simulink model "trackVehicleNewVer6b_Encoders_DR_GNC2"  (R2018a)
settings: Solver=ode45  StartTime=0.0  StopTime=300  FixedStep=0.1  RelTol=1e-3  EnableMultiTasking=on
PreLoadFcn:
  | RTWConfigurationCB('preloadfcn', bdroot);
InitFcn:
  | parameterVehicle
  | parameterGNC
StartFcn:
  | start
StopFcn:
  | stop
  | myStopFcn2sim(xActEst,yActEst,X_array,Y_array,rp1,rp2)
values from neighbouring files (symbols this model uses):
  b = 0.32    [parameterVehicle.m]
  bDR = 1*b    [parameterGNC.m]
  dcArrayC = [-100  -60 0  60  100]    [parameterGNC.m]
  dcArrayL = [-100 ... (first row only)    [parameterVehicle.m]
  dcArrayR = [-100 ... (first row only)    [parameterVehicle.m]
  eTick = 4300    [parameterVehicle.m]
  eTickDR = eTick    [parameterGNC.m]
  KP2 = 2    [parameterGNC.m]
  rl = 0.87*rNominal    (= 0.05366131029)    [parameterVehicle.m]
  rNominal = 0.061679667    [parameterVehicle.m]
  rNominalDR = rNominal    [parameterGNC.m]
  rp1 = 0.5    [parameterGNC.m]
  rp2 = 0.3    [parameterGNC.m]
  rr = 1.00*rNominal    (= 0.061679667)    [parameterVehicle.m]
  Tau1 = 0.001    [parameterGNC.m]
  Tau2 = 0.01    [parameterGNC.m]
  TauEncoderDR = 0.001    [parameterGNC.m]
  thetaIC = 0*(pi/180)    (= 0)    [parameterVehicle.m]
  Tsample = 1/10    (= 0.1)    [parameterGNC.m]
  TsampleEncoder = 1/10    (= 0.1)    [parameterVehicle.m]
  TsampleEncoderDR = TsampleEncoder    [parameterGNC.m]
  Vcom = 3*VmaxDR/4    [parameterGNC.m]
  wArrayC = [-VmaxDR, -Vmin, 0,  Vmin, VmaxDR]./rNominalDR    [parameterGNC.m]
  wArrayL = [-1.622403101 ... (first row only)    [parameterVehicle.m]
  wArrayR = [-1.288449612 ... (first row only)    [parameterVehicle.m]
  X_array = [1 2]    [parameterGNC.m]
  xIC = 0    [parameterVehicle.m]
  Y_array = [0 0]    [parameterGNC.m]
  yIC = 0    [parameterVehicle.m]
undefined symbols (not defined in the file or in its folder): DiscIntNeverNeededParam
libraries: simulink x13, robotlib x8, aerolibanimutils x1
CloseFcn:
  | rtwprivate ssgencode ModelCloseRequest track_vehicle6_v2
settings Model: Creator=Dogan  LastModifiedBy=askar
settings DataIOCC: LimitDataPoints=on  SaveFormat=Array
settings OptimizationCC: ExpressionDepthLimit=2147483647  InitFltsAndDblsToZero=on  LifeSpan=inf
settings DebuggingCC: SaveWithParameterizedLinksMsg=none  UnderspecifiedInitializationDetection=Classic  MergeDetectMultiDrivingBlocksExec=none  SignalResolutionControl=TryResolveAllWithWarning  SolverPrmCheckMsg=warning  MultiTaskDSMMsg=warning  MultiTaskCondExecSysMsg=none  FcnCallInpInsideContextMsg=warning  StateNameClashWarn=warning  SFUnexpectedBacktrackingDiag=warning  SFNoUnconditionalDefaultTransitionDiag=warning  SFExecutionAtInitializationDiag=none
settings HardwareCC: ProdBitPerLong=64  ProdLargestAtomicFloat=None  ProdHWDeviceType=Intel->x86-64  TargetHWDeviceType=32-bit Generic
settings ModelReferenceCC: PropagateSignalLabelsOutOfModel=off
settings SFSimCC: SimParseCustomCode=off
settings RTWCC: Description=Generic Real-Time Target
settings CodeAppCC: GenerateComments=off  SimulinkBlockComments=off
settings GRTTargetCC: TargetLangStandard=C89/C90 (ANSI)  GeneratePreprocessorConditionals=Disable all
settings ConfigComp: CovMetricSettings=dw  CovHtmlReporting=on  CovSaveCumulativeToWorkspaceVar=on  CovSaveSingleToWorkspaceVar=on  CovExternalEMLEnable=off

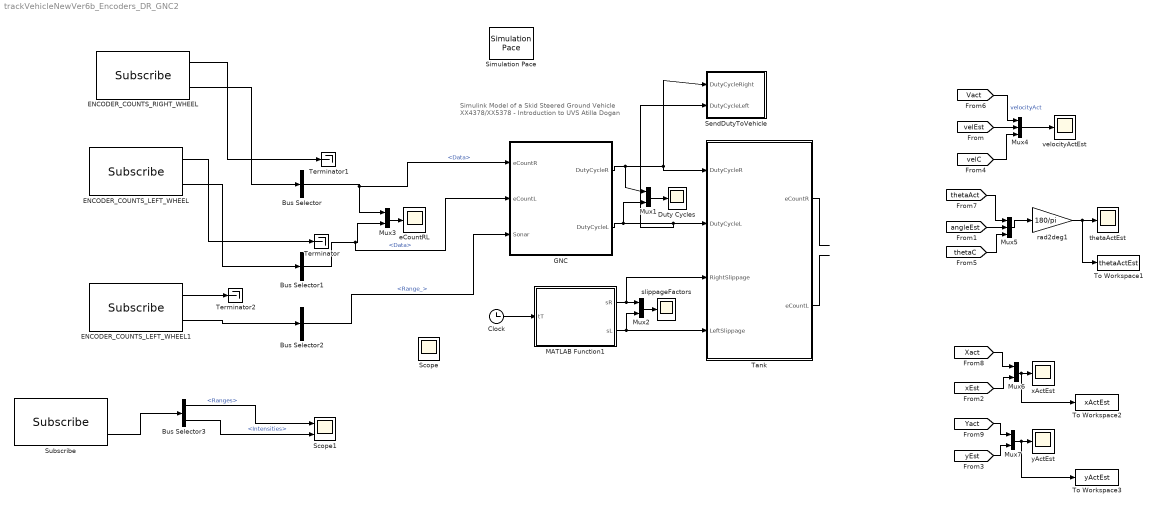
== system trackVehicleNewVer6b_Encoders_DR_GNC2 ==
  note: Simulink Model of a Skid Steered Ground Vehicle
      | XX4378/XX5378 - Introduction to UVS
      | Atilla Dogan
  Bus Selector : BusSelector  OutputSignals=Data
  Bus Selector1 : BusSelector  OutputSignals=Data
  Bus Selector2 : BusSelector  OutputSignals=Range_
  Bus Selector3 : BusSelector  OutputSignals=Ranges,Intensities
  Clock : Clock
  Duty Cycles : Scope
  ENCODER_COUNTS_LEFT_WHEEL : robotlib/Subscribe  SourceLibraryInfo=This block requires Robotics System Toolbox  topicSource=Select from ROS network  topic=/enco_L  messageType=std_msgs/Int16  sampleTime=-1  messageQueueLength=1
      settings: SourceProductBaseCode=RO
  ENCODER_COUNTS_LEFT_WHEEL1 : robotlib/Subscribe  SourceLibraryInfo=This block requires Robotics System Toolbox  topicSource=Select from ROS network  topic=/sonar  messageType=sensor_msgs/Range  sampleTime=-1  messageQueueLength=1
      settings: SourceProductBaseCode=RO
  ENCODER_COUNTS_RIGHT_WHEEL : robotlib/Subscribe  SourceLibraryInfo=This block requires Robotics System Toolbox  topicSource=Select from ROS network  topic=/enco_R  messageType=std_msgs/Int16  sampleTime=-1  messageQueueLength=1
      settings: SourceProductBaseCode=RO
  GNC : Subsystem
  MATLAB Function1 : MATLAB Function  TreatAsAtomicUnit=on
  Mux{1..3,6..7} (5 alike) : Mux  Inputs=2
  Mux4 : Mux  Inputs=3
  Mux5 : Mux  Inputs=3
  Scope : Scope
  Scope1 : Scope  NumInputPorts=2
  SendDutyToVehicle : Subsystem
  Simulation Pace : aerolibanimutils/Simulation Pace  SimulationPace=1  SleepMode=MATLAB Thread  OutputPaceError=off  SampleTime=1/30
  Subscribe : robotlib/Subscribe  SourceLibraryInfo=This block requires Robotics System Toolbox  topicSource=Select from ROS network  topic=/scan  messageType=sensor_msgs/LaserScan  sampleTime=-1  messageQueueLength=1
      settings: SourceProductBaseCode=RO
  Tank : Subsystem
  Terminator : Terminator
  Terminator1 : Terminator
  Terminator2 : Terminator
  To Workspace1 : ToWorkspace  VariableName=thetaActEst  SaveFormat=Structure With Time  SampleTime=-1
  To Workspace2 : ToWorkspace  VariableName=xActEst  SaveFormat=Structure With Time  SampleTime=-1
  To Workspace3 : ToWorkspace  VariableName=yActEst  SaveFormat=Structure With Time  SampleTime=-1
  eCountRL : Scope
  rad2deg1 : Gain  Gain=180/pi
  slippageFactors : Scope
  thetaActEst : Scope
  velocityActEst : Scope
  xActEst : Scope
  yActEst : Scope
  wires:
  MATLAB Function1/1(sR) -> Mux2/1, Tank/3(RightSlippage)
  MATLAB Function1/2(sL) -> Mux2/2, Tank/4(LeftSlippage)
  Clock/1 -> MATLAB Function1/1(tT)
  [Vact] -> Mux4/1  "velocityAct"
  GNC/1(DutyCycleR) -> Mux1/1, SendDutyToVehicle/1(DutyCycleRight), Tank/1(DutyCycleR)
  GNC/2(DutyCycleL) -> SendDutyToVehicle/2(DutyCycleLeft), Tank/2(DutyCycleL), Mux1/2
  Mux2/1 -> slippageFactors/1
  Mux1/1 -> Duty Cycles/1
  Tank/1(eCountR) -> ?
  Tank/2(eCountL) -> ?
  Mux4/1 -> velocityActEst/1
  [velEst] -> Mux4/2
  rad2deg1/1 -> To Workspace1/1, thetaActEst/1
  [thetaAct] -> Mux5/1
  Mux5/1 -> rad2deg1/1
  [angleEst] -> Mux5/2
  [Xact] -> Mux6/1
  [Yact] -> Mux7/1
  [xEst] -> Mux6/2
  Mux6/1 -> To Workspace2/1, xActEst/1
  Mux7/1 -> To Workspace3/1, yActEst/1
  [yEst] -> Mux7/2
  [velC] -> Mux4/3
  [thetaC] -> Mux5/3
  ENCODER_COUNTS_LEFT_WHEEL/1 -> Terminator/1
  ENCODER_COUNTS_RIGHT_WHEEL/2 -> Bus Selector/1
  ENCODER_COUNTS_RIGHT_WHEEL/1 -> Terminator1/1
  ENCODER_COUNTS_LEFT_WHEEL/2 -> Bus Selector1/1
  Bus Selector/1 -> GNC/1(eCountR), Mux3/1  "<Data>"
  Bus Selector1/1 -> GNC/2(eCountL), Mux3/2  "<Data>"
  Mux3/1 -> eCountRL/1
  ENCODER_COUNTS_LEFT_WHEEL1/2 -> Bus Selector2/1
  ENCODER_COUNTS_LEFT_WHEEL1/1 -> Terminator2/1
  Bus Selector2/1 -> GNC/3("Sonar ")  "<Range_>"
  Subscribe/2 -> Bus Selector3/1
  Bus Selector3/1 -> Scope1/1  "<Ranges>"
  Bus Selector3/2 -> Scope1/2  "<Intensities>"

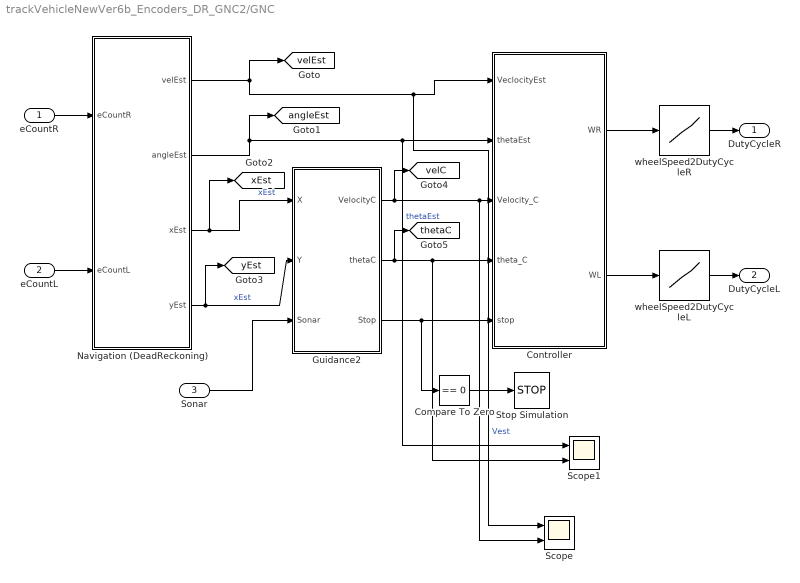
== system trackVehicleNewVer6b_Encoders_DR_GNC2/GNC ==
  eCountR : Inport
  eCountL : Inport  Port=2
  "Sonar " : Inport  Port=3
  Compare To Zero : simulink/Logic and Bit Operations/Compare To Zero  relop===  OutDataTypeStr=boolean
  Controller : Subsystem
  Guidance2 : Subsystem
  Navigation (DeadReckoning) : Subsystem
  Scope : Scope  NumInputPorts=2
  Scope1 : Scope  NumInputPorts=2
  Stop Simulation : Stop
  wheelSpeed2DutyCycleL : Lookup  InputValues=wArrayC  Table=dcArrayC  LookUpMeth=Interpolation-Use End Values
  wheelSpeed2DutyCycleR : Lookup  InputValues=wArrayC  Table=dcArrayC  LookUpMeth=Interpolation-Use End Values
  DutyCycleR : Outport
  DutyCycleL : Outport  Port=2
  tag scope: angleEst=global, thetaC=global, velC=global, velEst=global, xEst=global, yEst=global
  wires:
  Guidance2/3(Stop) -> Compare To Zero/1, Controller/5(stop)
  Controller/1(WR) -> wheelSpeed2DutyCycleR/1
  Navigation (DeadReckoning)/4(yEst) -> [yEst], Guidance2/2(Y)  "xEst"
  Navigation (DeadReckoning)/3(xEst) -> Guidance2/1(X), [xEst]  "xEst"
  Navigation (DeadReckoning)/2(angleEst) -> Scope1/1, Controller/2(thetaEst), [angleEst]  "thetaEst"
  Navigation (DeadReckoning)/1(velEst) -> Scope/1, Controller/1(VeclocityEst), [velEst]  "Vest"
  eCountL/1 -> Navigation (DeadReckoning)/2(eCountL)
  eCountR/1 -> Navigation (DeadReckoning)/1(eCountR)
  Guidance2/1(VelocityC) -> Scope/2, Controller/3(Velocity_C), [velC]
  Guidance2/2(thetaC) -> Scope1/2, Controller/4(theta_C), [thetaC]
  wheelSpeed2DutyCycleR/1 -> DutyCycleR/1
  Controller/2(WL) -> wheelSpeed2DutyCycleL/1
  wheelSpeed2DutyCycleL/1 -> DutyCycleL/1
  Compare To Zero/1 -> Stop Simulation/1
  "Sonar "/1 -> Guidance2/3("Sonar ")

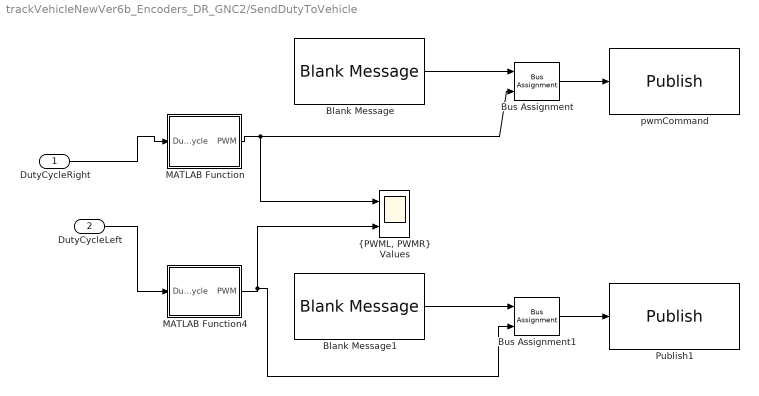
== system trackVehicleNewVer6b_Encoders_DR_GNC2/SendDutyToVehicle ==
  DutyCycleRight : Inport
  DutyCycleLeft : Inport  Port=2
  Blank Message : robotlib/Blank Message  SourceLibraryInfo=This block requires Robotics System Toolbox  messageType=std_msgs/Int16  SampleTime=inf
      settings: SourceProductBaseCode=RO
  Blank Message1 : robotlib/Blank Message  SourceLibraryInfo=This block requires Robotics System Toolbox  messageType=std_msgs/Int16  SampleTime=inf
      settings: SourceProductBaseCode=RO
  Bus Assignment : BusAssignment  AssignedSignals=Data
  Bus Assignment1 : BusAssignment  AssignedSignals=Data
  MATLAB Function : MATLAB Function  TreatAsAtomicUnit=on
  MATLAB Function4 : MATLAB Function  TreatAsAtomicUnit=on
  Publish1 : robotlib/Publish  SourceLibraryInfo=This block requires Robotics System Toolbox  topicSource=Select from ROS network  topic=/pwm_cmd_l  messageType=std_msgs/Int16  messageQueueLength=1
      settings: SourceProductBaseCode=RO
  pwmCommand : robotlib/Publish  SourceLibraryInfo=This block requires Robotics System Toolbox  topicSource=Select from ROS network  topic=/pwm_cmd_r  messageType=std_msgs/Int16  messageQueueLength=1
      settings: SourceProductBaseCode=RO
  "{PWML, PWMR} Values" : Scope  NumInputPorts=2
  wires:
  DutyCycleLeft/1 -> MATLAB Function4/1(DutyCycle)
  DutyCycleRight/1 -> MATLAB Function/1(DutyCycle)
  Blank Message/1 -> Bus Assignment/1
  MATLAB Function4/1(PWM) -> Bus Assignment1/2, "{PWML, PWMR} Values"/2
  MATLAB Function/1(PWM) -> Bus Assignment/2, "{PWML, PWMR} Values"/1
  Bus Assignment/1 -> pwmCommand/1
  Bus Assignment1/1 -> Publish1/1
  Blank Message1/1 -> Bus Assignment1/1

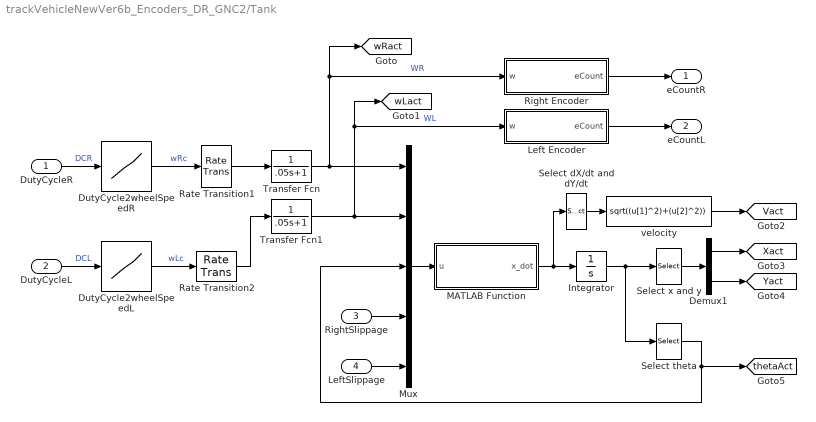
== system trackVehicleNewVer6b_Encoders_DR_GNC2/Tank ==
  DutyCycleR : Inport
  DutyCycleL : Inport  Port=2
  RightSlippage : Inport  Port=3
  LeftSlippage : Inport  Port=4
  Demux1 : Demux  Outputs=2
  DutyCycle2wheelSpeedL : Lookup  InputValues=dcArrayL  Table=wArrayL  LookUpMeth=Interpolation-Use End Values
  DutyCycle2wheelSpeedR : Lookup  InputValues=dcArrayR  Table=wArrayR  LookUpMeth=Interpolation-Use End Values
  Integrator : Integrator  InitialCondition=[xIC; yIC ; thetaIC]
  Left Encoder : Subsystem
  MATLAB Function : MATLAB Function  TreatAsAtomicUnit=on
  Mux : Mux  Inputs=5
  Rate Transition1 : RateTransition
  Rate Transition2 : RateTransition
  Right Encoder : Subsystem
  Select dX/dt and dY/dt : Selector  InputPortWidth=3  IndexOptions=Index vector (dialog)  Indices=[1 2]  OutputSizes=1
  Select theta : Selector  InputPortWidth=3  IndexOptions=Index vector (dialog)  Indices=3  OutputSizes=1
  Select x and y : Selector  InputPortWidth=3  IndexOptions=Index vector (dialog)  Indices=[1 2]  OutputSizes=1
  Transfer Fcn : TransferFcn  Denominator=[.05 1]
  Transfer Fcn1 : TransferFcn  Denominator=[.05 1]
  velocity : Fcn  Expr=sqrt((u[1]^2)+(u[2]^2))
  eCountR : Outport
  eCountL : Outport  Port=2
  tag scope: Vact=global, Xact=global, Yact=global, thetaAct=global, wLact=global, wRact=global
  wires:
  DutyCycleL/1 -> DutyCycle2wheelSpeedL/1  "DCL"
  DutyCycleR/1 -> DutyCycle2wheelSpeedR/1  "DCR"
  DutyCycle2wheelSpeedL/1 -> Rate Transition2/1  "wLc"
  DutyCycle2wheelSpeedR/1 -> Rate Transition1/1  "wRc"
  Rate Transition2/1 -> Transfer Fcn1/1
  Rate Transition1/1 -> Transfer Fcn/1
  Demux1/2 -> [Yact]
  Demux1/1 -> [Xact]
  Select x and y/1 -> Demux1/1
  velocity/1 -> [Vact]
  Select dX/dt and dY/dt/1 -> velocity/1
  MATLAB Function/1(x_dot) -> Integrator/1, Select dX/dt and dY/dt/1
  Select theta/1 -> [thetaAct], Mux/3
  Transfer Fcn/1 -> [wRact], Right Encoder/1(w), Mux/1  "WR"
  LeftSlippage/1 -> Mux/5
  RightSlippage/1 -> Mux/4
  Mux/1 -> MATLAB Function/1(u)
  Integrator/1 -> Select theta/1, Select x and y/1
  Transfer Fcn1/1 -> [wLact], Left Encoder/1(w), Mux/2  "WL"
  Left Encoder/1(eCount) -> eCountL/1
  Right Encoder/1(eCount) -> eCountR/1

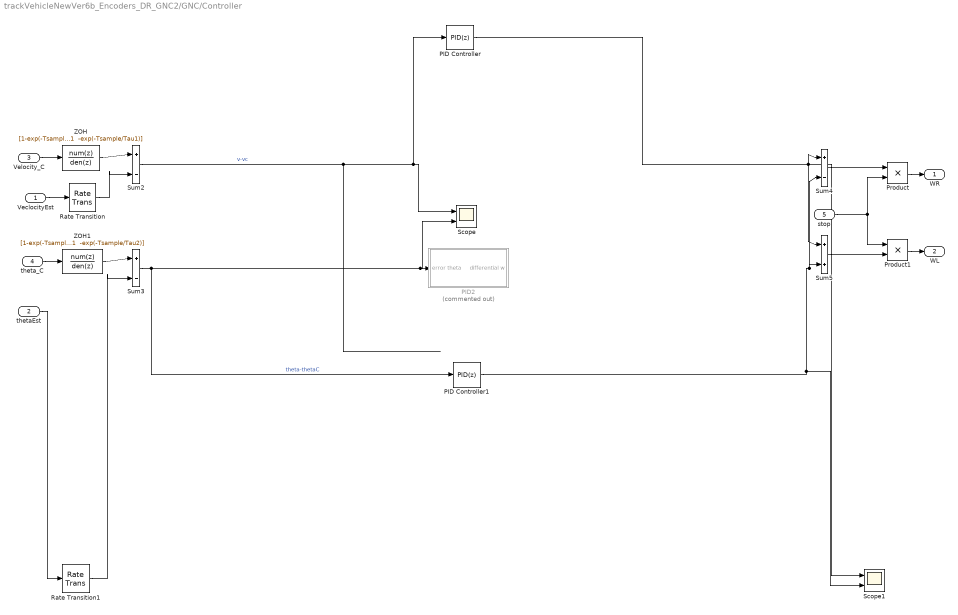
== system trackVehicleNewVer6b_Encoders_DR_GNC2/GNC/Controller ==
  VeclocityEst : Inport
  thetaEst : Inport  Port=2
  Velocity_C : Inport  Port=3
  theta_C : Inport  Port=4
  stop : Inport  Port=5
  PID Controller : simulink/Continuous/PID Controller  Controller=PID  TimeDomain=Discrete-time  SampleTime=-1  IntegratorMethod=Forward Euler  FilterMethod=Forward Euler  Form=Parallel  UseFilter=off  ControllerParametersSource=internal  P=2  I=7.0932  D=0.01  N=100  InitialConditionSource=internal  InitialConditionForIntegrator=0  InitialConditionForFilter=0  ExternalReset=none  LimitOutput=off  UpperSaturationLimit=inf  LowerSaturationLimit=-inf  LinearizeAsGain=on  AntiWindupMode=none  Kb=1  TrackingMode=off  Kt=1  PParamMin=[]  PParamMax=[]  IParamMin=[]  IParamMax=[]  DParamMin=[]  DParamMax=[]  NParamMin=[]  NParamMax=[]  KbParamMin=[]  KbParamMax=[]  KtParamMin=[]  KtParamMax=[]  POutMin=[]  POutMax=[]  IOutMin=[]  IOutMax=[]  DOutMin=[]  DOutMax=[]  NOutMin=[]  NOutMax=[]  KbOutMin=[]  KbOutMax=[]  KtOutMin=[]  KtOutMax=[]  IntegratorOutMin=[]  IntegratorOutMax=[]  FilterOutMin=[]  FilterOutMax=[]  SumOutMin=[]  SumOutMax=[]  SumI1OutMin=[]  SumI1OutMax=[]  SumI2OutMin=[]  SumI2OutMax=[]  SumI3OutMin=[]  SumI3OutMax=[]  SumDOutMin=[]  SumDOutMax=[]  SaturationOutMin=[]  SaturationOutMax=[]  IntegratorContinuousStateAttributes=''  IntegratorStateMustResolveToSignalObject=off  IntegratorRTWStateStorageClass=Auto  FilterContinuousStateAttributes=''  FilterStateMustResolveToSignalObject=off  FilterRTWStateStorageClass=Auto  DifferentiatorICPrevScaledInput=0  DifferentiatorOutMin=[]  DifferentiatorOutMax=[]  FilterDiffOutCoefMin=[]  FilterDiffOutCoefMax=[]  SumDenOutMin=[]  SumDenOutMax=[]  SumNumOutMin=[]  SumNumOutMax=[]  ReciprocalOutMin=[]  ReciprocalOutMax=[]  DivideOutMin=[]  DivideOutMax=[]  TunerSelectOption=Frequency Response Based
  PID Controller1 : simulink/Continuous/PID Controller  Controller=PID  TimeDomain=Discrete-time  SampleTime=-1  IntegratorMethod=Forward Euler  FilterMethod=Forward Euler  Form=Parallel  UseFilter=off  ControllerParametersSource=internal  P=6.4  I=1.2  D=1.8  N=100  InitialConditionSource=internal  InitialConditionForIntegrator=0  InitialConditionForFilter=0  ExternalReset=none  LimitOutput=off  UpperSaturationLimit=inf  LowerSaturationLimit=-inf  LinearizeAsGain=on  AntiWindupMode=none  Kb=1  TrackingMode=off  Kt=1  PParamMin=[]  PParamMax=[]  IParamMin=[]  IParamMax=[]  DParamMin=[]  DParamMax=[]  NParamMin=[]  NParamMax=[]  KbParamMin=[]  KbParamMax=[]  KtParamMin=[]  KtParamMax=[]  POutMin=[]  POutMax=[]  IOutMin=[]  IOutMax=[]  DOutMin=[]  DOutMax=[]  NOutMin=[]  NOutMax=[]  KbOutMin=[]  KbOutMax=[]  KtOutMin=[]  KtOutMax=[]  IntegratorOutMin=[]  IntegratorOutMax=[]  FilterOutMin=[]  FilterOutMax=[]  SumOutMin=[]  SumOutMax=[]  SumI1OutMin=[]  SumI1OutMax=[]  SumI2OutMin=[]  SumI2OutMax=[]  SumI3OutMin=[]  SumI3OutMax=[]  SumDOutMin=[]  SumDOutMax=[]  SaturationOutMin=[]  SaturationOutMax=[]  IntegratorContinuousStateAttributes=''  IntegratorStateMustResolveToSignalObject=off  IntegratorRTWStateStorageClass=Auto  FilterContinuousStateAttributes=''  FilterStateMustResolveToSignalObject=off  FilterRTWStateStorageClass=Auto  DifferentiatorICPrevScaledInput=0  DifferentiatorOutMin=[]  DifferentiatorOutMax=[]  FilterDiffOutCoefMin=[]  FilterDiffOutCoefMax=[]  SumDenOutMin=[]  SumDenOutMax=[]  SumNumOutMin=[]  SumNumOutMax=[]  ReciprocalOutMin=[]  ReciprocalOutMax=[]  DivideOutMin=[]  DivideOutMax=[]  TunerSelectOption=Frequency Response Based
  PID2 : Subsystem  Commented=on
  Product : Product  RndMeth=Zero
  Product1 : Product  RndMeth=Zero
  Rate Transition : RateTransition  Deterministic=off
  Rate Transition1 : RateTransition  Deterministic=off
  Scope : Scope  NumInputPorts=2
  Scope1 : Scope  NumInputPorts=2
  Sum2 : Sum  Inputs=|+|-|  SampleTime=Tsample
  Sum3 : Sum  Inputs=|+|-|  SampleTime=Tsample
  Sum4 : Sum  Inputs=+|-
  Sum5 : Sum  Inputs=+|+
  ZOH : DiscreteTransferFcn  Numerator=[1-exp(-Tsample/Tau1)]  Denominator="[1  -exp(-Tsample/Tau1)]"  SampleTime=Tsample
  ZOH1 : DiscreteTransferFcn  Numerator=[1-exp(-Tsample/Tau2)]  Denominator="[1  -exp(-Tsample/Tau2)]"  SampleTime=Tsample
  WR : Outport
  WL : Outport  Port=2
  wires:
  Product1/1 -> WL/1
  Product/1 -> WR/1
  Sum5/1 -> Product1/2
  stop/1 -> Product/2, Product1/1
  Sum4/1 -> Product/1
  theta_C/1 -> ZOH1/1
  thetaEst/1 -> Rate Transition1/1
  Velocity_C/1 -> ZOH/1
  VeclocityEst/1 -> Rate Transition/1
  Sum2/1 -> PID Controller/1, Scope/1  "v-vc"
  Sum3/1 -> PID Controller1/1, Scope/2, PID2/1(error theta)  "theta-thetaC"
  ZOH/1 -> Sum2/1
  Rate Transition/1 -> Sum2/2
  ZOH1/1 -> Sum3/1
  Rate Transition1/1 -> Sum3/2
  PID Controller/1 -> Scope1/1, Sum5/1, Sum4/1
  PID Controller1/1 -> Sum5/2, Sum4/2, Scope1/2

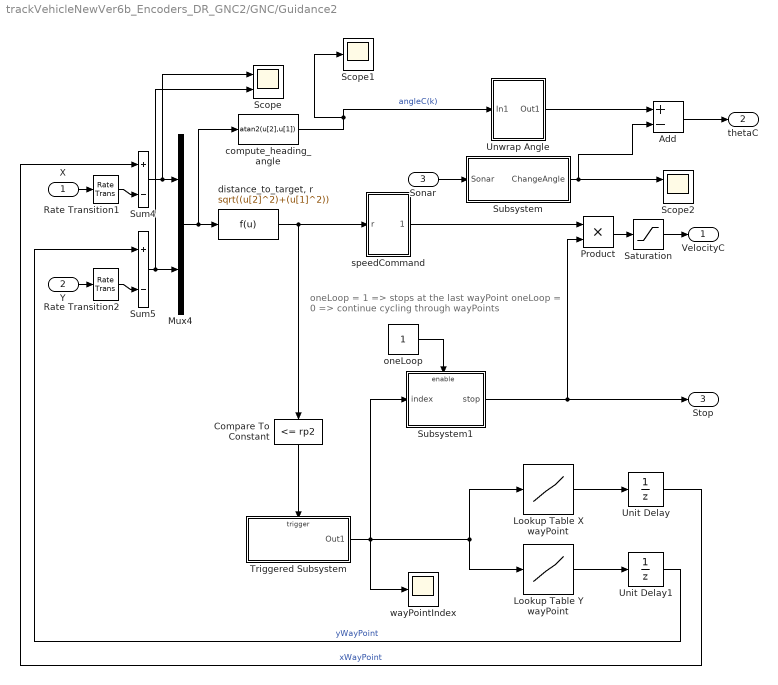
== system trackVehicleNewVer6b_Encoders_DR_GNC2/GNC/Guidance2 ==
  note: oneLoop = 1 => stops at the last wayPoint
      | oneLoop = 0 => continue cycling through wayPoints
  X : Inport
  Y : Inport  Port=2
  "Sonar " : Inport  Port=3
  Add : Sum  Inputs=+-
  Compare To Constant : simulink/Logic and Bit Operations/Compare To Constant  relop=<=  const=rp2  OutDataTypeStr=uint8  ZeroCross=off
  Lookup Table X wayPoint : Lookup  InputValues=[1:length(X_array)]  Table=X_array  LookUpMeth=Interpolation-Use End Values  OutDataTypeStr=double
  Lookup Table Y wayPoint : Lookup  InputValues=[1:length(Y_array)]  Table=Y_array  LookUpMeth=Interpolation-Use End Values  OutDataTypeStr=double
  Mux4 : Mux  Inputs=2
  Product : Product  RndMeth=Zero
  Rate Transition1 : RateTransition
  Rate Transition2 : RateTransition
  Saturation : Saturate  UpperLimit=Vcom  LowerLimit=0  SampleTime=Tsample
  Scope : Scope  NumInputPorts=2
  Scope1 : Scope
  Scope2 : Scope  NumInputPorts=2
  Subsystem : Subsystem
  Subsystem1 : Subsystem
  Sum4 : Sum  Inputs=|+|-|
  Sum5 : Sum  Inputs=|+|-|
  Triggered Subsystem : Subsystem  TreatAsAtomicUnit=on
  Unit Delay : UnitDelay  SampleTime=Tsample
  Unit Delay1 : UnitDelay  SampleTime=Tsample
  Unwrap Angle : Subsystem
  compute_heading_angle : Fcn  Expr=atan2(u[2],u[1])  SampleTime=Tsample
  "distance_to_target, r" : Fcn  Expr=sqrt((u[2]^2)+(u[1]^2))  SampleTime=Tsample
  oneLoop : Constant  OutDataTypeStr=uint32  SampleTime=Tsample
  speedCommand : Subsystem
  wayPointIndex : Scope
  VelocityC : Outport
  thetaC : Outport  Port=2
  Stop : Outport  Port=3
  wires:
  speedCommand/1(Vdes) -> Product/1
  compute_heading_angle/1 -> Scope1/1, Unwrap Angle/1(In1)  "angleC(k)"
  Sum4/1 -> Scope/1, Mux4/1
  "distance_to_target, r"/1 -> Compare To Constant/1, speedCommand/1(r)
  Mux4/1 -> "distance_to_target, r"/1, compute_heading_angle/1
  Lookup Table X wayPoint/1 -> Unit Delay/1
  Lookup Table Y wayPoint/1 -> Unit Delay1/1
  X/1 -> Rate Transition1/1
  Y/1 -> Rate Transition2/1
  Sum5/1 -> Mux4/2, Scope/2
  Compare To Constant/1 -> Triggered Subsystem/Trigger
  Triggered Subsystem/1(Out1) -> Subsystem1/1(index), wayPointIndex/1, Lookup Table X wayPoint/1, Lookup Table Y wayPoint/1
  Unit Delay/1 -> Sum4/1  "xWayPoint"
  Unit Delay1/1 -> Sum5/1  "yWayPoint"
  Saturation/1 -> VelocityC/1
  Rate Transition1/1 -> Sum4/2
  Rate Transition2/1 -> Sum5/2
  Product/1 -> Saturation/1
  Subsystem1/1(stop) -> Product/2, Stop/1
  oneLoop/1 -> Subsystem1/Enable
  "Sonar "/1 -> Subsystem/1("Sonar ")
  Unwrap Angle/1(Out1) -> Add/1
  Add/1 -> thetaC/1
  Subsystem/1("ChangeAngle ") -> Add/2, Scope2/1

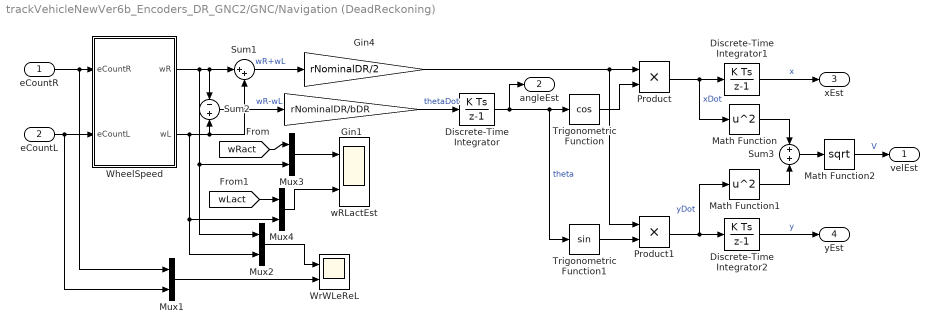
== system trackVehicleNewVer6b_Encoders_DR_GNC2/GNC/Navigation (DeadReckoning) ==
  eCountR : Inport
  eCountL : Inport  Port=2
  Discrete-Time Integrator : DiscreteIntegrator  SampleTime=TsampleEncoderDR  ICPrevOutput=DiscIntNeverNeededParam  ICPrevScaledInput=DiscIntNeverNeededParam
  Discrete-Time Integrator1 : DiscreteIntegrator  SampleTime=TsampleEncoderDR  ICPrevOutput=DiscIntNeverNeededParam  ICPrevScaledInput=DiscIntNeverNeededParam
  Discrete-Time Integrator2 : DiscreteIntegrator  SampleTime=TsampleEncoderDR  ICPrevOutput=DiscIntNeverNeededParam  ICPrevScaledInput=DiscIntNeverNeededParam
  Gin1 : Gain  Gain=rNominalDR/bDR  OutDataTypeStr=double
  Gin4 : Gain  Gain=rNominalDR/2  OutDataTypeStr=double
  Math Function : Math  Operator=square  SaturateOnIntegerOverflow=on
  Math Function1 : Math  Operator=square  SaturateOnIntegerOverflow=on
  Math Function2 : Math  Operator=sqrt  OutputSignalType=real  SaturateOnIntegerOverflow=on
  Mux{1..4} (4 alike) : Mux  Inputs=2
  Product : Product  RndMeth=Zero
  Product1 : Product  RndMeth=Zero
  Sum1 : Sum  Inputs=|++
  Sum2 : Sum  Inputs=-|+
  Sum3 : Sum  Inputs=+|+
  Trigonometric Function : Trigonometry  Operator=cos  OutputSignalType=real
  Trigonometric Function1 : Trigonometry  OutputSignalType=real
  WheelSpeed : Subsystem
  WrWLeReL : Scope  NumInputPorts=2
  wRLactEst : Scope  NumInputPorts=2
  velEst : Outport
  angleEst : Outport  Port=2
  xEst : Outport  Port=3
  yEst : Outport  Port=4
  wires:
  [wLact] -> Mux4/1
  [wRact] -> Mux3/1
  Mux4/1 -> wRLactEst/2
  Mux3/1 -> wRLactEst/1
  Mux2/1 -> WrWLeReL/1
  Mux1/1 -> WrWLeReL/2
  Math Function2/1 -> velEst/1  "V"
  Sum3/1 -> Math Function2/1
  Math Function1/1 -> Sum3/2
  Math Function/1 -> Sum3/1
  Discrete-Time Integrator2/1 -> yEst/1  "y"
  Discrete-Time Integrator1/1 -> xEst/1  "x"
  Product1/1 -> Math Function1/1, Discrete-Time Integrator2/1  "yDot"
  Product/1 -> Math Function/1, Discrete-Time Integrator1/1  "xDot"
  Trigonometric Function1/1 -> Product1/2
  Gin4/1 -> Product1/1, Product/1
  Trigonometric Function/1 -> Product/2
  Discrete-Time Integrator/1 -> angleEst/1, Trigonometric Function1/1, Trigonometric Function/1  "theta"
  Gin1/1 -> Discrete-Time Integrator/1  "thetaDot"
  Sum2/1 -> Gin1/1  "wR-wL"
  Sum1/1 -> Gin4/1  "wR+wL"
  WheelSpeed/1(wR) -> Mux3/2, Mux2/1, Sum2/1, Sum1/1
  WheelSpeed/2(wL) -> Mux4/2, Mux2/2, Sum2/2, Sum1/2
  eCountL/1 -> Mux1/2, WheelSpeed/2(eCountL)
  eCountR/1 -> Mux1/1, WheelSpeed/1(eCountR)

== system trackVehicleNewVer6b_Encoders_DR_GNC2/Tank/Left Encoder ==
  w : Inport
  Rate Transition1 : RateTransition
  WheelAngleL : Integrator
  angle2tick2 : Gain  Gain=eTick*rNominal  OutDataTypeStr=int16  SampleTime=TsampleEncoder
  eCount : Outport
  wires:
  WheelAngleL/1 -> Rate Transition1/1  "gammaL"
  w/1 -> WheelAngleL/1
  angle2tick2/1 -> eCount/1  "eCountL"
  Rate Transition1/1 -> angle2tick2/1

== system trackVehicleNewVer6b_Encoders_DR_GNC2/Tank/Right Encoder ==
  w : Inport
  Rate Transition1 : RateTransition
  WheelAngleR : Integrator
  angle2tick1 : Gain  Gain=eTick*rNominal  OutDataTypeStr=int16  SampleTime=TsampleEncoder
  eCount : Outport
  wires:
  WheelAngleR/1 -> Rate Transition1/1  "gammaR"
  w/1 -> WheelAngleR/1
  angle2tick1/1 -> eCount/1  "eCountR"
  Rate Transition1/1 -> angle2tick1/1

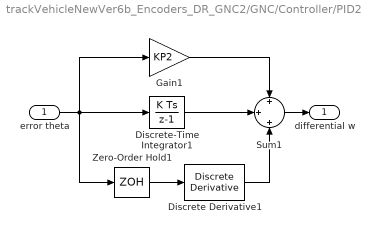
== system trackVehicleNewVer6b_Encoders_DR_GNC2/GNC/Controller/PID2 ==
  error theta : Inport
  Discrete Derivative1 : simulink/Discrete/Discrete Derivative  gainval=KD2  ICPrevScaledInput=0.0  InputProcessing=Inherited  OutMin=[]  OutMax=[]  OutDataType=sfix(16)  OutScaling=2^-10  DoSatur=off
  Discrete-Time Integrator1 : DiscreteIntegrator  gainval=KI2  SampleTime=Tsample  ICPrevOutput=DiscIntNeverNeededParam  ICPrevScaledInput=DiscIntNeverNeededParam
  Gain1 : Gain  Gain=KP2  SampleTime=Tsample
  Sum1 : Sum  Inputs=+|+|+
  Zero-Order Hold1 : ZeroOrderHold  SampleTime=Tsample
  differential w : Outport
  wires:
  Discrete Derivative1/1 -> Sum1/3
  Zero-Order Hold1/1 -> Discrete Derivative1/1
  error theta/1 -> Gain1/1, Discrete-Time Integrator1/1, Zero-Order Hold1/1
  Discrete-Time Integrator1/1 -> Sum1/2
  Gain1/1 -> Sum1/1
  Sum1/1 -> differential w/1

== system trackVehicleNewVer6b_Encoders_DR_GNC2/GNC/Guidance2/Subsystem ==
  "Sonar " : Inport
  Delay : Delay  DelayLength=1
  MATLAB Function : MATLAB Function  TreatAsAtomicUnit=on
  "ChangeAngle " : Outport  OutDataTypeStr=double
  wires:
  MATLAB Function/1(changeAngle) -> Delay/1, "ChangeAngle "/1
  "Sonar "/1 -> MATLAB Function/1(sonar)
  Delay/1 -> MATLAB Function/2(changeAnglePrev)

== system trackVehicleNewVer6b_Encoders_DR_GNC2/GNC/Guidance2/Subsystem1 ==
  note: NAND = TRUE
      | if at least one input is FALSE
  index : Inport
  Enable : EnablePort
  Compare To Constant1 : simulink/Logic and Bit Operations/Compare To Constant  relop===  const=1  OutDataTypeStr=uint8  ZeroCross=off
  Compare To Constant2 : simulink/Logic and Bit Operations/Compare To Constant  relop===  const=length(X_array)  OutDataTypeStr=uint8  ZeroCross=off
  Logical Operator1 : Logic  Operator=NAND  IconShape=distinctive  AllPortsSameDT=off  OutDataTypeStr=boolean
  Triggered Subsystem2 : Subsystem  TreatAsAtomicUnit=on
  stop : Outport  OutputWhenDisabled=reset  InitialOutput=[1]
  wires:
  Logical Operator1/1 -> stop/1
  index/1 -> Compare To Constant1/1, Compare To Constant2/1
  Compare To Constant1/1 -> Logical Operator1/1
  Triggered Subsystem2/1(Out1) -> Logical Operator1/2
  Compare To Constant2/1 -> Triggered Subsystem2/Trigger

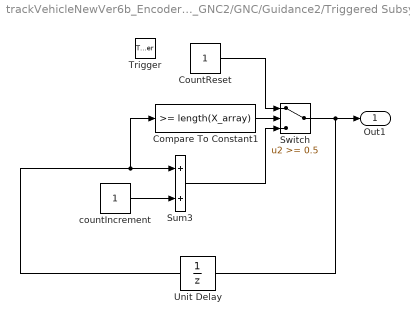
== system trackVehicleNewVer6b_Encoders_DR_GNC2/GNC/Guidance2/Triggered Subsystem ==
  Trigger : TriggerPort  VariantControl=(inherit)
  Compare To Constant1 : simulink/Logic and Bit Operations/Compare To Constant  relop=>=  const=length(X_array)  OutDataTypeStr=uint8  ZeroCross=off
  CountReset : Constant  OutDataTypeStr=uint32  SampleTime=-1
  Sum3 : Sum  OutDataTypeStr=uint32
  Switch : Switch  Threshold=0.5
  Unit Delay : UnitDelay  InitialCondition=1  SampleTime=-1
  countIncrement : Constant  OutDataTypeStr=uint32  SampleTime=-1
  Out1 : Outport  OutDataTypeStr=uint32  InitialOutput=1
  wires:
  countIncrement/1 -> Sum3/2
  Unit Delay/1 -> Sum3/1, Compare To Constant1/1
  Compare To Constant1/1 -> Switch/2
  Switch/1 -> Out1/1, Unit Delay/1
  CountReset/1 -> Switch/1
  Sum3/1 -> Switch/3

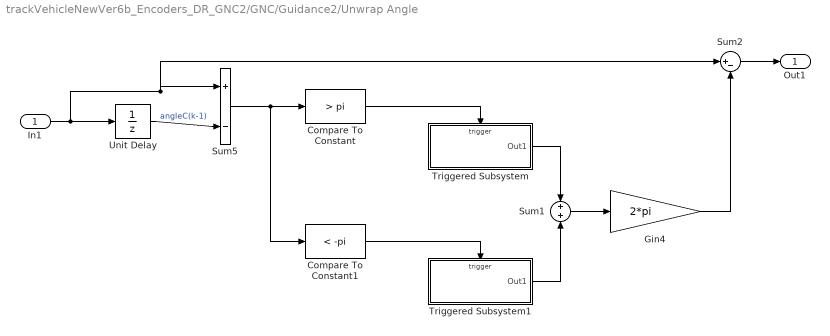
== system trackVehicleNewVer6b_Encoders_DR_GNC2/GNC/Guidance2/Unwrap Angle ==
  In1 : Inport
  Compare To Constant : simulink/Logic and Bit Operations/Compare To Constant  relop=>  const=pi  OutDataTypeStr=uint8  ZeroCross=off
  Compare To Constant1 : simulink/Logic and Bit Operations/Compare To Constant  relop=<  const=-pi  OutDataTypeStr=uint8  ZeroCross=off
  Gin4 : Gain  Gain=2*pi  OutDataTypeStr=double  SampleTime=Tsample
  Sum1 : Sum  Inputs=+|+
  Sum2 : Sum  Inputs=|+-
  Sum5 : Sum  Inputs=|+|-|
  Triggered Subsystem : Subsystem  TreatAsAtomicUnit=on
  Triggered Subsystem1 : Subsystem  TreatAsAtomicUnit=on
  Unit Delay : UnitDelay  SampleTime=Tsample
  Out1 : Outport
  wires:
  In1/1 -> Unit Delay/1, Sum5/1, Sum2/1
  Unit Delay/1 -> Sum5/2  "angleC(k-1)"
  Sum5/1 -> Compare To Constant/1, Compare To Constant1/1
  Compare To Constant1/1 -> Triggered Subsystem1/Trigger
  Compare To Constant/1 -> Triggered Subsystem/Trigger
  Triggered Subsystem/1(Out1) -> Sum1/1
  Triggered Subsystem1/1(Out1) -> Sum1/2
  Sum1/1 -> Gin4/1
  Sum2/1 -> Out1/1
  Gin4/1 -> Sum2/2

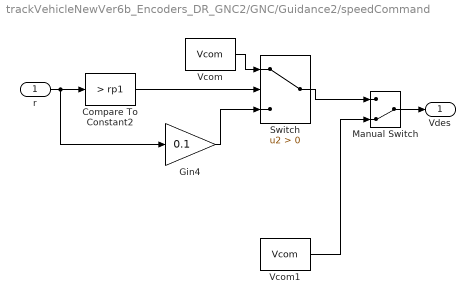
== system trackVehicleNewVer6b_Encoders_DR_GNC2/GNC/Guidance2/speedCommand ==
  r : Inport
  Compare To Constant2 : simulink/Logic and Bit Operations/Compare To Constant  relop=>  const=rp1  OutDataTypeStr=uint8  ZeroCross=off
  Gin4 : Gain  Gain=0.1  SampleTime=Tsample
  Manual Switch : ManualSwitch  CurrentSetting=0
  Switch : Switch  Criteria=u2 > Threshold
  Vcom : Constant  Value=Vcom  SampleTime=Tsample
  Vcom1 : Constant  Value=Vcom  SampleTime=Tsample
  Vdes : Outport
  wires:
  Compare To Constant2/1 -> Switch/2
  Vcom/1 -> Switch/1
  Vcom1/1 -> Manual Switch/2
  Switch/1 -> Manual Switch/1
  Gin4/1 -> Switch/3
  r/1 -> Compare To Constant2/1, Gin4/1
  Manual Switch/1 -> Vdes/1

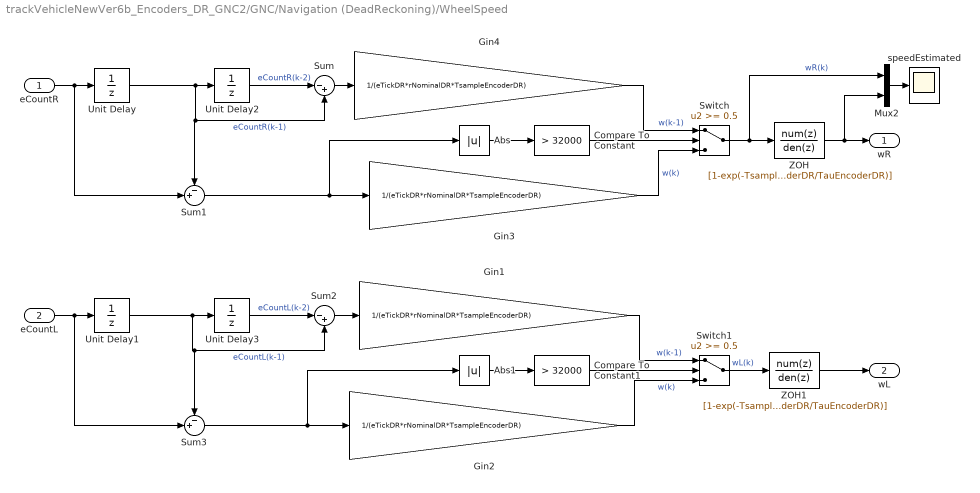
== system trackVehicleNewVer6b_Encoders_DR_GNC2/GNC/Navigation (DeadReckoning)/WheelSpeed ==
  eCountR : Inport
  eCountL : Inport  Port=2
  Abs : Abs
  Abs1 : Abs
  Compare To Constant : simulink/Logic and Bit Operations/Compare To Constant  relop=>  const=32000  OutDataTypeStr=uint8  ZeroCross=off
  Compare To Constant1 : simulink/Logic and Bit Operations/Compare To Constant  relop=>  const=32000  OutDataTypeStr=uint8  ZeroCross=off
  Gin{1..4} (4 alike) : Gain  Gain=1/(eTickDR*rNominalDR*TsampleEncoderDR)  OutDataTypeStr=double  SampleTime=TsampleEncoderDR
  Mux2 : Mux  Inputs=2
  Sum : Sum  Inputs=|-+
  Sum1 : Sum  Inputs=-+|
  Sum2 : Sum  Inputs=|-+
  Sum3 : Sum  Inputs=-+|
  Switch : Switch  Threshold=0.5
  Switch1 : Switch  Threshold=0.5
  Unit Delay{,1..3} (4 alike) : UnitDelay  SampleTime=TsampleEncoderDR
  ZOH : DiscreteTransferFcn  Numerator=[1-exp(-TsampleEncoderDR/TauEncoderDR)]  Denominator="[1  -exp(-TsampleEncoderDR/TauEncoderDR)]"  SampleTime=TsampleEncoderDR
  ZOH1 : DiscreteTransferFcn  Numerator=[1-exp(-TsampleEncoderDR/TauEncoderDR)]  Denominator="[1  -exp(-TsampleEncoderDR/TauEncoderDR)]"  SampleTime=TsampleEncoderDR
  speedEstimated : Scope
  wR : Outport
  wL : Outport  Port=2
  wires:
  Mux2/1 -> speedEstimated/1
  ZOH1/1 -> wL/1
  ZOH/1 -> Mux2/2, wR/1
  Switch1/1 -> ZOH1/1  "wL(k)"
  Switch/1 -> Mux2/1, ZOH/1  "wR(k)"
  Compare To Constant1/1 -> Switch1/2
  Abs1/1 -> Compare To Constant1/1
  Gin2/1 -> Switch1/3  "w(k)"
  Gin1/1 -> Switch1/1  "w(k-1)"
  Sum3/1 -> Gin2/1, Abs1/1
  Sum2/1 -> Gin1/1
  Unit Delay3/1 -> Sum2/1  "eCountL(k-2)"
  Unit Delay1/1 -> Unit Delay3/1, Sum2/2, Sum3/1  "eCountL(k-1)"
  eCountL/1 -> Unit Delay1/1, Sum3/2
  Compare To Constant/1 -> Switch/2
  Abs/1 -> Compare To Constant/1
  Gin3/1 -> Switch/3  "w(k)"
  Gin4/1 -> Switch/1  "w(k-1)"
  Sum1/1 -> Gin3/1, Abs/1
  Sum/1 -> Gin4/1
  Unit Delay2/1 -> Sum/1  "eCountR(k-2)"
  Unit Delay/1 -> Sum1/1, Sum/2, Unit Delay2/1  "eCountR(k-1)"
  eCountR/1 -> Sum1/2, Unit Delay/1

== system trackVehicleNewVer6b_Encoders_DR_GNC2/GNC/Guidance2/Subsystem1/Triggered Subsystem2 ==
  Trigger : TriggerPort  VariantControl=(inherit)
  Constant : Constant  OutDataTypeStr=uint32  SampleTime=-1
  Out1 : Outport  OutDataTypeStr=uint32  InitialOutput=0
  wires:
  Constant/1 -> Out1/1

== system trackVehicleNewVer6b_Encoders_DR_GNC2/GNC/Guidance2/Unwrap Angle/Triggered Subsystem ==
  Trigger : TriggerPort  VariantControl=(inherit)
  Sum3 : Sum  OutDataTypeStr=int32
  Unit Delay : UnitDelay  SampleTime=-1
  countIncrement : Constant  OutDataTypeStr=int32  SampleTime=-1
  Out1 : Outport  OutDataTypeStr=int32  InitialOutput=0
  wires:
  countIncrement/1 -> Sum3/2
  Unit Delay/1 -> Sum3/1
  Sum3/1 -> Out1/1, Unit Delay/1

== system trackVehicleNewVer6b_Encoders_DR_GNC2/GNC/Guidance2/Unwrap Angle/Triggered Subsystem1 ==
  Trigger : TriggerPort  VariantControl=(inherit)
  Sum3 : Sum  Inputs=+-  OutDataTypeStr=int32
  Unit Delay : UnitDelay  SampleTime=-1
  countIncrement : Constant  OutDataTypeStr=int32  SampleTime=-1
  Out1 : Outport  OutDataTypeStr=int32  InitialOutput=0
  wires:
  Sum3/1 -> Out1/1, Unit Delay/1
  Unit Delay/1 -> Sum3/1
  countIncrement/1 -> Sum3/2

== matlab function trackVehicleNewVer6b_Encoders_DR_GNC2/Tank/MATLAB Function ==
  data: u input; x_dot output; b parameter; rr parameter; rl parameter
function x_dot = fcn(u,b,rr,rl)
%#codegen

wr = u(1);
wl = u(2);
theta = u(3);
sr = u(4);
sl = u(5);
x_dot = [((1-sl)*rl*wl + (1-sr)*rr*wr)*cos(theta)/2;
         ((1-sl)*rl*wl + (1-sr)*rr*wr)*sin(theta)/2;
         ((1-sl)*rl*wl - (1-sr)*rr*wr)/b];

== matlab function trackVehicleNewVer6b_Encoders_DR_GNC2/GNC/Guidance2/Subsystem/MATLAB Function ==
  data: sonar input; changeAngle output double; changeAnglePrev input
function changeAngle = fcn(sonar, changeAnglePrev)
gain = 45/sonar;
if gain > 0.6
    changeAngle = double(gain * 22/7 * 1/3);
    
else
    if changeAnglePrev > 0
        changeAngle = changeAnglePrev - 0.1;
    else
        changeAngle = 0.0;
    end
end

== matlab function trackVehicleNewVer6b_Encoders_DR_GNC2/MATLAB Function1 ==
  data: tT input; sR output; sL output
function [sR,sL] = slipFnc(tT)
%#codegen

% tT  : time
% sR  : slippage on Right Track
% sL  : slippage on Left Track

% initialization
sR=0;sL=0;

% if tT > 38 && tT < 43
% %     sR=0.2;
%     sL=0.2;
% end
% %

== matlab function trackVehicleNewVer6b_Encoders_DR_GNC2/SendDutyToVehicle/MATLAB Function ==
  data: DutyCycle input; PWM output
function PWM = fcn(DutyCycle)
  

        PWM = int16(DutyCycle/100 * 255);
    end

== matlab function trackVehicleNewVer6b_Encoders_DR_GNC2/SendDutyToVehicle/MATLAB Function4 ==
  data: DutyCycle input; PWM output
function PWM = fcn(DutyCycle)

    PWM = int16(DutyCycle/100 * 255);
